simulink model "UAVNLCL_MOD"  (R2023a)
settings: Solver=ode45  StartTime=0.0  StopTime=1  RelTol=1e-3  EnableMultiTasking=on
values from neighbouring files (symbols this model uses):
  K = Klqr    [Calculos00_OriginalIgnacio.m]    (also in PI_4_OBSOLETE_TestingPredictedController.m = state2k(state); PI_5_PIofVariousPredictedController.m = reshape(DATA(index,3:12), 2, 5); PI_6_Tracker_bigGuy.m = zeros(2,5); PI_9_playground_state2k.m = state2k(state))
  W = 2.5    [Calculos00_OriginalIgnacio.m]    (also in Calculos02_Vnoladetrim.m; Calculos03_TablaTrimados.m; GenerateDataset_v0.m; PI_0_OnlyOneController_V20.m)
  x0 = [-1 0 -0.5 -0.5 0]    [BackUp_Simulation_002.mat]    (also in Calculos00_OriginalIgnacio.m = [0,deltaAoA,0,0,0]; Calculos02_Vnoladetrim.m = [1, 0, 0, 0, 0]; GenerateDataset_v0.m = [-1,0,0,0,0]'; PI_0_OnlyOneController_V20.m = [-1,0,0,0,0]')
  XCG = 0.33    [Calculos00_OriginalIgnacio.m]    (also in Calculos02_Vnoladetrim.m; Calculos03_TablaTrimados.m; GenerateDataset_v0.m; PI_0_OnlyOneController_V20.m)
undefined symbols (not defined in the file or in its folder): Utrim, Xtrim
settings Model: Creator=Ignacio  LastModifiedBy=ignac
settings SolverCC: AlgebraicLoopSolver=TrustRegion
settings DataIOCC: ExternalInput=[0 0.369809473744665 -0.0760167506859634 0.299999999999976]  InitialState=[]  LimitDataPoints=on  SaveFormat=Array  SignalLoggingSaveFormat=ModelDataLogs  ReturnWorkspaceOutputs=off
settings OptimizationCC: DefaultParameterBehavior=Inlined  BufferReuse=off  ExpressionDepthLimit=2147483647  LifeSpan=inf
settings DebuggingCC: UnderspecifiedInitializationDetection=Classic  MergeDetectMultiDrivingBlocksExec=none  FcnCallInpInsideContextMsg=warning  UnconnectedInputMsg=warning  UnconnectedOutputMsg=warning  UnconnectedLineMsg=warning  StateNameClashWarn=warning  InitInArrayFormatMsg=none  SFUnexpectedBacktrackingDiag=warning  SFNoUnconditionalDefaultTransitionDiag=warning  SFExecutionAtInitializationDiag=none  ArithmeticOperatorsInVariantConditions=warning
settings HardwareCC: ProdBitPerPointer=32  ProdBitPerSizeT=32  ProdBitPerPtrDiffT=32  ProdLargestAtomicFloat=None  ProdIntDivRoundTo=Undefined  ProdEndianess=Unspecified  ProdWordSize=32  ProdHWDeviceType=32-bit Generic
settings ModelReferenceCC: EnableRefExpFcnMdlSchedulingChecks=on  PropagateSignalLabelsOutOfModel=off
settings SFSimCC: SimUseLocalCustomCode=off  CustomCodeUndefinedFunction=UseInterfaceOnly
settings RTWCC: RTWUseLocalCustomCode=off
settings CodeAppCC: StateflowObjectComments=on
settings GRTTargetCC: TargetLangStandard=C89/C90 (ANSI)
settings ConfigComp: CovMetricSettings=dw  CovSaveCumulativeToWorkspaceVar=on  CovSaveSingleToWorkspaceVar=on  CovExternalEMLEnable=off

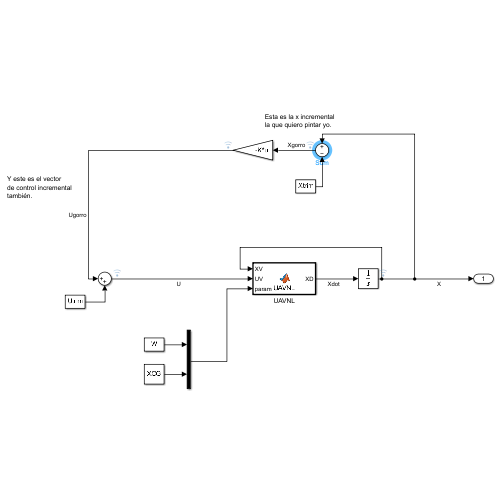
[thumbnail: Simulink's stored preview of the top-level diagram]
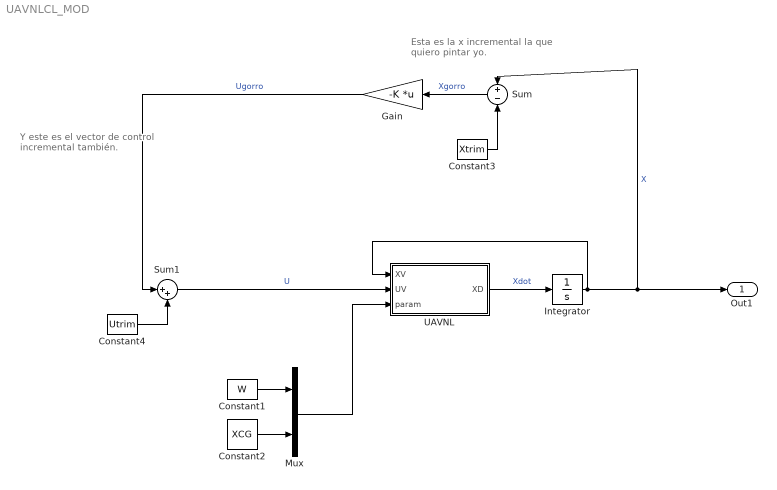
== system UAVNLCL_MOD ==
  note: Y este es el vector
      | de control incremental
      | también.
  note: Esta es la x incremental
      | la que quiero pintar yo.
  Constant1 : Constant  Value=W
  Constant2 : Constant  Value=XCG
  Constant3 : Constant  Value=Xtrim
  Constant4 : Constant  Value=Utrim
  Gain : Gain  Gain=-K  Multiplication=Matrix(K*u)
  Integrator : Integrator  InitialCondition=Xtrim+x0
  Mux : Mux  Inputs=2
  Sum : Sum  Inputs=+-
  Sum1 : Sum  Inputs=|++
  UAVNL : MATLAB Function  TreatAsAtomicUnit=on
  Out1 : Outport
  wires:
  UAVNL/1(XD) -> Integrator/1  "Xdot"
  Integrator/1 -> Sum/1, Out1/1, UAVNL/1(XV)  "X"
  Constant1/1 -> Mux/1
  Constant2/1 -> Mux/2
  Mux/1 -> UAVNL/3(param)
  Sum/1 -> Gain/1  "Xgorro"
  Constant3/1 -> Sum/2
  Sum1/1 -> UAVNL/2(UV)  "U"
  Gain/1 -> Sum1/1  "Ugorro"
  Constant4/1 -> Sum1/2

== matlab function UAVNLCL_MOD/UAVNL ==
  data: XV input; XD output; UV input; param input
function XD = UAVNL(XV,UV,param)

% DATOS DE LA AERONAVE

S = 0.4121;                 % Superficie alar (m^2)
C = 0.2192;                 % Cuerda media aerodinámica (m)
% MASA = 2.5;                 % Masa (Kg)
XCGR = 0.33;                % Posición de referencia del CG (xcg/c)
IP = 0.156794;              % Momento de inercia (Kg*m^2)
% d = 1.225;                  % Densidad (Kg/m^3)
G = 9.8;                    % Gravedad (m/s^2)
% XCG = .33;                  % CG no coincide con el de referencia

% Derivadas de estabilidad y control adimensionales

CLalpha0=0.405;    
CLalpha=5.379292;
CLq=11.133615;
CD0=0.0277;
CDalpha=0.14897;
CDalpha2=0.9848;
Cm0=0.0418;     
Cmalpha=-6.0; %-1.812981 más inestable en cabeceo
Cmalphadot=-7.0;
Cmde=-1.552;
Cmq=-18.422237;

% Variables de estado

VT = XV(1);	    % Velocidad aerodinámica
ALPHA = XV(2);	% Angulo de ataque
THETA = XV(3);  % Angulo de asiento
Q = XV(4);	    % Velocidad angular de cabeceo
H = XV(5);      % Altura

% Variables de control

Dt = UV(1);	    % Acelerador
De = UV(2);	    % Deflexión del timón de profundidad

% Parameters

MASA = param(1);    % Masa
XCG = param(2);     % Posición del centro de gravedad (adim, xcg/c)

% Densidad a la altura H

d = density(H);

% Algunos calculos previos

U = VT*cos(ALPHA);	    % Componentes de la velocidad en ejes cuerpo
W = VT*sin(ALPHA);	

PDS = 0.5*d*(VT^2)*S;   % (Presión dinámica) * (Superficie alar)

% Parametros Grupo Motopropulsor

Dh = 0.254;             % Diametro de la helice (m)
REVmax = 222;           % Revoluciones máximas del motor (rev/s)

CT0 = 0.13805;          % Coeficientes de traccion
CTj = -0.2049;
REV = REVmax*Dt;        % Revoluciones instantáneas
J = VT/(REV*Dh);        % Coeficiente de velocidad
C_T = CT0+CTj*J;        % Coef de tracción
T = C_T*d*REV^2*Dh^4;   % Traccion

% coeficientes adimensionales de fuerzas y momentos (ejes viento)

CLT=CLalpha0+CLalpha*ALPHA+CLq*Q*C*0.5/VT;         
CDT=CD0+CDalpha*ALPHA+CDalpha2*ALPHA^2;  
CZ=-CDT*sin(ALPHA)-CLT*cos(ALPHA); % Cz en ejes cuerpo para añadir despues el efecto del centro de gravedad
CmT=Cm0+(Cmalpha*ALPHA)+(Cmde*De)+(CZ*(XCG-XCGR))+(C*0.5*Cmq*Q/VT); % Falta la componente alphadot,la añadiremos despues

% Fuerzas aerodinámicas

L = CLT*PDS;
D = CDT*PDS;

% Sistema de ecuaciones diferenciales de la dinámica del vuelo


UDOT = -Q*W+(T-MASA*G*sin(THETA)-D*cos(ALPHA)+L*sin(ALPHA))/MASA;
WDOT = Q*U+(MASA*G*cos(THETA)-D*sin(ALPHA)-L*cos(ALPHA))/MASA;
ALPHADOT = (U*WDOT-W*UDOT)/VT^2;
CmT = CmT + Cmalphadot*C/(2*VT)*ALPHADOT; % Completamos Cm
QDOT = CmT*PDS*C/IP;

VTDOT=(U*UDOT+W*WDOT)/VT;

% Vector con las derivadas de las variables de estado

XD = zeros(5,1);
XD(1) = VTDOT;
XD(2) = ALPHADOT;
XD(3) = Q;
XD(4) = QDOT;
XD(5) = VT*sin(THETA-ALPHA);
